simulink library "Enrg_conv_El_to_Mec_Bosch"  (R2016a)
settings: Solver=ode1  StartTime=0.0  StopTime=Inf  FixedStep=0.001  RelTol=1e-3
undefined symbols (not defined in the file): drvEmot_RefTqeMOT, FirstDrivenAxle_FirstDrivenAxleNoOfEmot, FMIKit, SecondDrivenAxle_SecondDrivenAxleNoOfEmot
libraries: Enrg_conv_El_to_Mec_Bosch x13, Electrical_converter x8
(part 3 of 5)

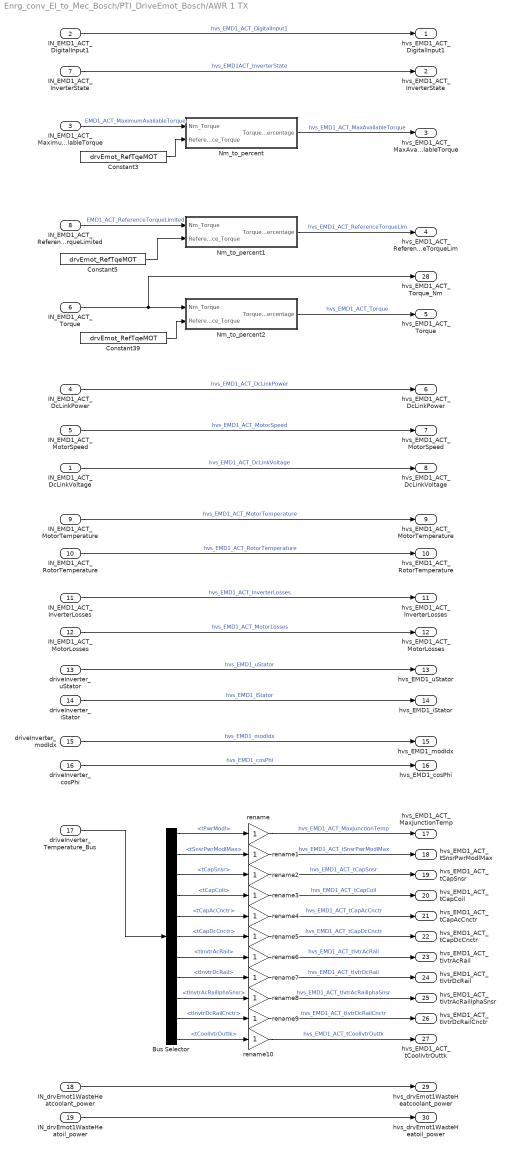
== system Enrg_conv_El_to_Mec_Bosch/PTI_DriveEmot_Bosch/AWR 1 TX ==
  IN_EMD1_ACT_DcLinkVoltage : Inport
  IN_EMD1_ACT_DigitalInput1 : Inport  Port=2
  IN_EMD1_ACT_MaximumAvailableTorque : Inport  Port=3
  IN_EMD1_ACT_DcLinkPower : Inport  Port=4
  IN_EMD1_ACT_MotorSpeed : Inport  Port=5
  IN_EMD1_ACT_Torque : Inport  Port=6
  IN_EMD1_ACT_InverterState : Inport  Port=7
  IN_EMD1_ACT_ReferenceTorqueLimited : Inport  Port=8
  IN_EMD1_ACT_MotorTemperature : Inport  Port=9
  IN_EMD1_ACT_RotorTemperature : Inport  Port=10
  IN_EMD1_ACT_InverterLosses : Inport  Port=11
  IN_EMD1_ACT_MotorLosses : Inport  Port=12
  driveInverter_uStator : Inport  Port=13
  driveInverter_iStator : Inport  Port=14
  driveInverter_modIdx : Inport  Port=15
  driveInverter_cosPhi : Inport  Port=16
  driveInverter_Temperature_Bus : Inport  Port=17
  IN_drvEmot1WasteHeatcoolant_power : Inport  Port=18
  IN_drvEmot1WasteHeatoil_power : Inport  Port=19
  Bus Selector : BusSelector  OutputSignals=tPwrModl,tSnsrPwrModlMax,tCapSnsr,tCapCoil,tCapAcCnctr,tCapDcCnctr,tInvtrAcRail,tInvtrDcRail,tInvtrAcRailIphaSnsr,tInvtrDcRailCnctr,tCoolIvtrOuttk
  Constant3 : Constant  Value=drvEmot_RefTqeMOT
  Constant39 : Constant  Value=drvEmot_RefTqeMOT
  Constant5 : Constant  Value=drvEmot_RefTqeMOT
  Nm_to_percent : Subsystem
  Nm_to_percent1 : Subsystem
  Nm_to_percent2 : Subsystem
  rename{,1..10} (11 alike) : Gain
  hvs_EMD1_ACT_DigitalInput1 : Outport
  hvs_EMD1_ACT_InverterState : Outport  Port=2
  hvs_EMD1_ACT_MaxAvailableTorque : Outport  Port=3
  hvs_EMD1_ACT_ReferenceTorqueLim : Outport  Port=4
  hvs_EMD1_ACT_Torque : Outport  Port=5
  hvs_EMD1_ACT_DcLinkPower : Outport  Port=6
  hvs_EMD1_ACT_MotorSpeed : Outport  Port=7
  hvs_EMD1_ACT_DcLinkVoltage : Outport  Port=8
  hvs_EMD1_ACT_MotorTemperature : Outport  Port=9
  hvs_EMD1_ACT_RotorTemperature : Outport  Port=10
  hvs_EMD1_ACT_InverterLosses : Outport  Port=11
  hvs_EMD1_ACT_MotorLosses : Outport  Port=12
  hvs_EMD1_uStator : Outport  Port=13
  hvs_EMD1_iStator : Outport  Port=14
  hvs_EMD1_modIdx : Outport  Port=15
  hvs_EMD1_cosPhi : Outport  Port=16
  hvs_EMD1_ACT_MaxJunctionTemp : Outport  Port=17
  hvs_EMD1_ACT_tSnsrPwrModlMax : Outport  Port=18
  hvs_EMD1_ACT_tCapSnsr : Outport  Port=19
  hvs_EMD1_ACT_tCapCoil : Outport  Port=20
  hvs_EMD1_ACT_tCapAcCnctr : Outport  Port=21
  hvs_EMD1_ACT_tCapDcCnctr : Outport  Port=22
  hvs_EMD1_ACT_tIvtrAcRail : Outport  Port=23
  hvs_EMD1_ACT_tIvtrDcRail : Outport  Port=24
  hvs_EMD1_ACT_tIvtrAcRailIphaSnsr : Outport  Port=25
  hvs_EMD1_ACT_tIvtrDcRailCnctr : Outport  Port=26
  hvs_EMD1_ACT_tCoolIvtrOuttk : Outport  Port=27
  hvs_EMD1_ACT_Torque_Nm : Outport  Port=28
  hvs_drvEmot1WasteHeatcoolant_power : Outport  Port=29
  hvs_drvEmot1WasteHeatoil_power : Outport  Port=30
  wires:
  Constant5/1 -> Nm_to_percent1/2(Reference_Torque)
  IN_EMD1_ACT_ReferenceTorqueLimited/1 -> Nm_to_percent1/1(Nm_Torque)  "EMD1_ACT_ReferenceTorqueLimited"
  IN_EMD1_ACT_InverterState/1 -> hvs_EMD1_ACT_InverterState/1  "hvs_EMD1ACT_InverterState"
  IN_EMD1_ACT_DcLinkPower/1 -> hvs_EMD1_ACT_DcLinkPower/1  "hvs_EMD1_ACT_DcLinkPower"
  IN_EMD1_ACT_DcLinkVoltage/1 -> hvs_EMD1_ACT_DcLinkVoltage/1  "hvs_EMD1_ACT_DcLinkVoltage"
  Nm_to_percent/1(Torque_Percentage) -> hvs_EMD1_ACT_MaxAvailableTorque/1  "hvs_EMD1_ACT_MaxAvailableTorque"
  Nm_to_percent1/1(Torque_Percentage) -> hvs_EMD1_ACT_ReferenceTorqueLim/1  "hvs_EMD1_ACT_ReferenceTorqueLim"
  IN_EMD1_ACT_MotorSpeed/1 -> hvs_EMD1_ACT_MotorSpeed/1  "hvs_EMD1_ACT_MotorSpeed"
  IN_EMD1_ACT_Torque/1 -> hvs_EMD1_ACT_Torque_Nm/1, Nm_to_percent2/1(Nm_Torque)
  IN_EMD1_ACT_MotorTemperature/1 -> hvs_EMD1_ACT_MotorTemperature/1  "hvs_EMD1_ACT_MotorTemperature"
  IN_EMD1_ACT_DigitalInput1/1 -> hvs_EMD1_ACT_DigitalInput1/1  "hvs_EMD1_ACT_DigitalInput1"
  IN_EMD1_ACT_MaximumAvailableTorque/1 -> Nm_to_percent/1(Nm_Torque)  "EMD1_ACT_MaximumAvailableTorque"
  Constant3/1 -> Nm_to_percent/2(Reference_Torque)
  Nm_to_percent2/1(Torque_Percentage) -> hvs_EMD1_ACT_Torque/1  "hvs_EMD1_ACT_Torque"
  Constant39/1 -> Nm_to_percent2/2(Reference_Torque)
  IN_EMD1_ACT_InverterLosses/1 -> hvs_EMD1_ACT_InverterLosses/1  "hvs_EMD1_ACT_InverterLosses"
  IN_EMD1_ACT_MotorLosses/1 -> hvs_EMD1_ACT_MotorLosses/1  "hvs_EMD1_ACT_MotorLosses"
  IN_EMD1_ACT_RotorTemperature/1 -> hvs_EMD1_ACT_RotorTemperature/1  "hvs_EMD1_ACT_RotorTemperature"
  driveInverter_uStator/1 -> hvs_EMD1_uStator/1  "hvs_EMD1_uStator"
  driveInverter_iStator/1 -> hvs_EMD1_iStator/1  "hvs_EMD1_iStator"
  driveInverter_Temperature_Bus/1 -> Bus Selector/1
  Bus Selector/1 -> rename/1  "<tPwrModl>"
  Bus Selector/2 -> rename1/1  "<tSnsrPwrModlMax>"
  Bus Selector/3 -> rename2/1  "<tCapSnsr>"
  Bus Selector/4 -> rename3/1  "<tCapCoil>"
  Bus Selector/5 -> rename4/1  "<tCapAcCnctr>"
  Bus Selector/6 -> rename5/1  "<tCapDcCnctr>"
  Bus Selector/7 -> rename6/1  "<tInvtrAcRail>"
  Bus Selector/8 -> rename7/1  "<tInvtrDcRail>"
  Bus Selector/9 -> rename8/1  "<tInvtrAcRailIphaSnsr>"
  Bus Selector/10 -> rename9/1  "<tInvtrDcRailCnctr>"
  Bus Selector/11 -> rename10/1  "<tCoolIvtrOuttk>"
  rename/1 -> hvs_EMD1_ACT_MaxJunctionTemp/1  "hvs_EMD1_ACT_MaxJunctionTemp"
  rename1/1 -> hvs_EMD1_ACT_tSnsrPwrModlMax/1  "hvs_EMD1_ACT_tSnsrPwrModlMax"
  rename2/1 -> hvs_EMD1_ACT_tCapSnsr/1  "hvs_EMD1_ACT_tCapSnsr"
  rename3/1 -> hvs_EMD1_ACT_tCapCoil/1  "hvs_EMD1_ACT_tCapCoil"
  rename4/1 -> hvs_EMD1_ACT_tCapAcCnctr/1  "hvs_EMD1_ACT_tCapAcCnctr"
  rename5/1 -> hvs_EMD1_ACT_tCapDcCnctr/1  "hvs_EMD1_ACT_tCapDcCnctr"
  rename6/1 -> hvs_EMD1_ACT_tIvtrAcRail/1  "hvs_EMD1_ACT_tIvtrAcRail"
  rename7/1 -> hvs_EMD1_ACT_tIvtrDcRail/1  "hvs_EMD1_ACT_tIvtrDcRail"
  rename8/1 -> hvs_EMD1_ACT_tIvtrAcRailIphaSnsr/1  "hvs_EMD1_ACT_tIvtrAcRailIphaSnsr"
  rename9/1 -> hvs_EMD1_ACT_tIvtrDcRailCnctr/1  "hvs_EMD1_ACT_tIvtrDcRailCnctr"
  rename10/1 -> hvs_EMD1_ACT_tCoolIvtrOuttk/1  "hvs_EMD1_ACT_tCoolIvtrOuttk"
  driveInverter_modIdx/1 -> hvs_EMD1_modIdx/1  "hvs_EMD1_modIdx"
  driveInverter_cosPhi/1 -> hvs_EMD1_cosPhi/1  "hvs_EMD1_cosPhi"
  IN_drvEmot1WasteHeatcoolant_power/1 -> hvs_drvEmot1WasteHeatcoolant_power/1
  IN_drvEmot1WasteHeatoil_power/1 -> hvs_drvEmot1WasteHeatoil_power/1

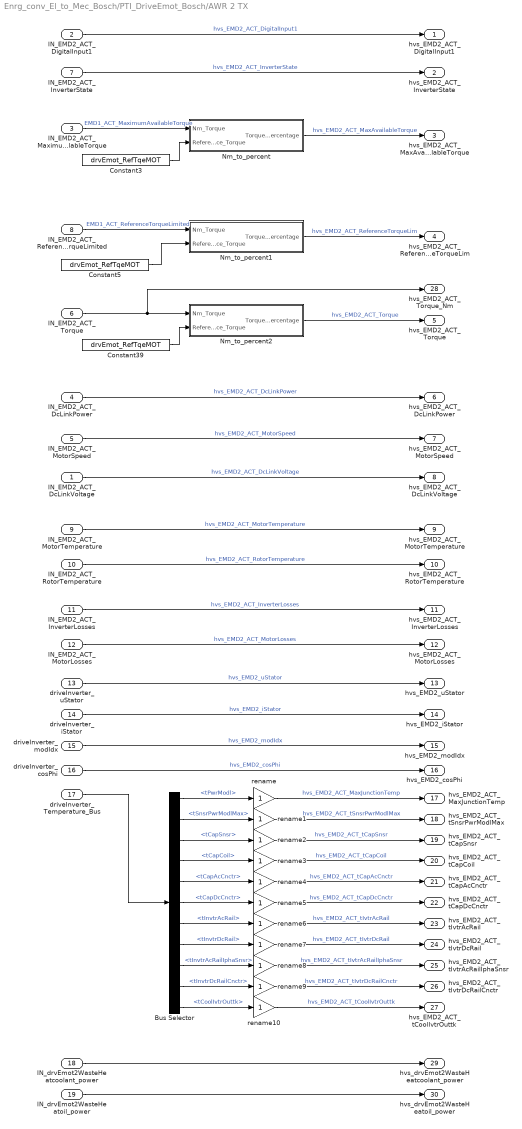
== system Enrg_conv_El_to_Mec_Bosch/PTI_DriveEmot_Bosch/AWR 2 TX ==
  IN_EMD2_ACT_DcLinkVoltage : Inport
  IN_EMD2_ACT_DigitalInput1 : Inport  Port=2
  IN_EMD2_ACT_MaximumAvailableTorque : Inport  Port=3
  IN_EMD2_ACT_DcLinkPower : Inport  Port=4
  IN_EMD2_ACT_MotorSpeed : Inport  Port=5
  IN_EMD2_ACT_Torque : Inport  Port=6
  IN_EMD2_ACT_InverterState : Inport  Port=7
  IN_EMD2_ACT_ReferenceTorqueLimited : Inport  Port=8
  IN_EMD2_ACT_MotorTemperature : Inport  Port=9
  IN_EMD2_ACT_RotorTemperature : Inport  Port=10
  IN_EMD2_ACT_InverterLosses : Inport  Port=11
  IN_EMD2_ACT_MotorLosses : Inport  Port=12
  driveInverter_uStator : Inport  Port=13
  driveInverter_iStator : Inport  Port=14
  driveInverter_modIdx : Inport  Port=15
  driveInverter_cosPhi : Inport  Port=16
  driveInverter_Temperature_Bus : Inport  Port=17
  IN_drvEmot2WasteHeatcoolant_power : Inport  Port=18
  IN_drvEmot2WasteHeatoil_power : Inport  Port=19
  Bus Selector : BusSelector  OutputSignals=tPwrModl,tSnsrPwrModlMax,tCapSnsr,tCapCoil,tCapAcCnctr,tCapDcCnctr,tInvtrAcRail,tInvtrDcRail,tInvtrAcRailIphaSnsr,tInvtrDcRailCnctr,tCoolIvtrOuttk
  Constant3 : Constant  Value=drvEmot_RefTqeMOT
  Constant39 : Constant  Value=drvEmot_RefTqeMOT
  Constant5 : Constant  Value=drvEmot_RefTqeMOT
  Nm_to_percent : Subsystem
  Nm_to_percent1 : Subsystem
  Nm_to_percent2 : Subsystem
  rename{,1..10} (11 alike) : Gain
  hvs_EMD2_ACT_DigitalInput1 : Outport
  hvs_EMD2_ACT_InverterState : Outport  Port=2
  hvs_EMD2_ACT_MaxAvailableTorque : Outport  Port=3
  hvs_EMD2_ACT_ReferenceTorqueLim : Outport  Port=4
  hvs_EMD2_ACT_Torque : Outport  Port=5
  hvs_EMD2_ACT_DcLinkPower : Outport  Port=6
  hvs_EMD2_ACT_MotorSpeed : Outport  Port=7
  hvs_EMD2_ACT_DcLinkVoltage : Outport  Port=8
  hvs_EMD2_ACT_MotorTemperature : Outport  Port=9
  hvs_EMD2_ACT_RotorTemperature : Outport  Port=10
  hvs_EMD2_ACT_InverterLosses : Outport  Port=11
  hvs_EMD2_ACT_MotorLosses : Outport  Port=12
  hvs_EMD2_uStator : Outport  Port=13
  hvs_EMD2_iStator : Outport  Port=14
  hvs_EMD2_modIdx : Outport  Port=15
  hvs_EMD2_cosPhi : Outport  Port=16
  hvs_EMD2_ACT_MaxJunctionTemp : Outport  Port=17
  hvs_EMD2_ACT_tSnsrPwrModlMax : Outport  Port=18
  hvs_EMD2_ACT_tCapSnsr : Outport  Port=19
  hvs_EMD2_ACT_tCapCoil : Outport  Port=20
  hvs_EMD2_ACT_tCapAcCnctr : Outport  Port=21
  hvs_EMD2_ACT_tCapDcCnctr : Outport  Port=22
  hvs_EMD2_ACT_tIvtrAcRail : Outport  Port=23
  hvs_EMD2_ACT_tIvtrDcRail : Outport  Port=24
  hvs_EMD2_ACT_tIvtrAcRailIphaSnsr : Outport  Port=25
  hvs_EMD2_ACT_tIvtrDcRailCnctr : Outport  Port=26
  hvs_EMD2_ACT_tCoolIvtrOuttk : Outport  Port=27
  hvs_EMD2_ACT_Torque_Nm : Outport  Port=28
  hvs_drvEmot2WasteHeatcoolant_power : Outport  Port=29
  hvs_drvEmot2WasteHeatoil_power : Outport  Port=30
  wires:
  Constant5/1 -> Nm_to_percent1/2(Reference_Torque)
  IN_EMD2_ACT_ReferenceTorqueLimited/1 -> Nm_to_percent1/1(Nm_Torque)  "EMD1_ACT_ReferenceTorqueLimited"
  IN_EMD2_ACT_InverterState/1 -> hvs_EMD2_ACT_InverterState/1  "hvs_EMD2_ACT_InverterState"
  IN_EMD2_ACT_DcLinkPower/1 -> hvs_EMD2_ACT_DcLinkPower/1  "hvs_EMD2_ACT_DcLinkPower"
  IN_EMD2_ACT_DcLinkVoltage/1 -> hvs_EMD2_ACT_DcLinkVoltage/1  "hvs_EMD2_ACT_DcLinkVoltage"
  Nm_to_percent/1(Torque_Percentage) -> hvs_EMD2_ACT_MaxAvailableTorque/1  "hvs_EMD2_ACT_MaxAvailableTorque"
  Nm_to_percent1/1(Torque_Percentage) -> hvs_EMD2_ACT_ReferenceTorqueLim/1  "hvs_EMD2_ACT_ReferenceTorqueLim"
  IN_EMD2_ACT_MotorSpeed/1 -> hvs_EMD2_ACT_MotorSpeed/1  "hvs_EMD2_ACT_MotorSpeed"
  IN_EMD2_ACT_Torque/1 -> hvs_EMD2_ACT_Torque_Nm/1, Nm_to_percent2/1(Nm_Torque)
  IN_EMD2_ACT_MotorTemperature/1 -> hvs_EMD2_ACT_MotorTemperature/1  "hvs_EMD2_ACT_MotorTemperature"
  IN_EMD2_ACT_DigitalInput1/1 -> hvs_EMD2_ACT_DigitalInput1/1  "hvs_EMD2_ACT_DigitalInput1"
  IN_EMD2_ACT_MaximumAvailableTorque/1 -> Nm_to_percent/1(Nm_Torque)  "EMD1_ACT_MaximumAvailableTorque"
  Constant3/1 -> Nm_to_percent/2(Reference_Torque)
  Nm_to_percent2/1(Torque_Percentage) -> hvs_EMD2_ACT_Torque/1  "hvs_EMD2_ACT_Torque"
  Constant39/1 -> Nm_to_percent2/2(Reference_Torque)
  IN_EMD2_ACT_InverterLosses/1 -> hvs_EMD2_ACT_InverterLosses/1  "hvs_EMD2_ACT_InverterLosses"
  IN_EMD2_ACT_MotorLosses/1 -> hvs_EMD2_ACT_MotorLosses/1  "hvs_EMD2_ACT_MotorLosses"
  IN_EMD2_ACT_RotorTemperature/1 -> hvs_EMD2_ACT_RotorTemperature/1  "hvs_EMD2_ACT_RotorTemperature"
  driveInverter_uStator/1 -> hvs_EMD2_uStator/1  "hvs_EMD2_uStator"
  driveInverter_iStator/1 -> hvs_EMD2_iStator/1  "hvs_EMD2_iStator"
  driveInverter_Temperature_Bus/1 -> Bus Selector/1
  Bus Selector/1 -> rename/1  "<tPwrModl>"
  Bus Selector/2 -> rename1/1  "<tSnsrPwrModlMax>"
  Bus Selector/3 -> rename2/1  "<tCapSnsr>"
  Bus Selector/4 -> rename3/1  "<tCapCoil>"
  Bus Selector/5 -> rename4/1  "<tCapAcCnctr>"
  Bus Selector/6 -> rename5/1  "<tCapDcCnctr>"
  Bus Selector/7 -> rename6/1  "<tInvtrAcRail>"
  Bus Selector/8 -> rename7/1  "<tInvtrDcRail>"
  Bus Selector/9 -> rename8/1  "<tInvtrAcRailIphaSnsr>"
  Bus Selector/10 -> rename9/1  "<tInvtrDcRailCnctr>"
  Bus Selector/11 -> rename10/1  "<tCoolIvtrOuttk>"
  rename/1 -> hvs_EMD2_ACT_MaxJunctionTemp/1  "hvs_EMD2_ACT_MaxJunctionTemp"
  rename1/1 -> hvs_EMD2_ACT_tSnsrPwrModlMax/1  "hvs_EMD2_ACT_tSnsrPwrModlMax"
  rename2/1 -> hvs_EMD2_ACT_tCapSnsr/1  "hvs_EMD2_ACT_tCapSnsr"
  rename3/1 -> hvs_EMD2_ACT_tCapCoil/1  "hvs_EMD2_ACT_tCapCoil"
  rename4/1 -> hvs_EMD2_ACT_tCapAcCnctr/1  "hvs_EMD2_ACT_tCapAcCnctr"
  rename5/1 -> hvs_EMD2_ACT_tCapDcCnctr/1  "hvs_EMD2_ACT_tCapDcCnctr"
  rename6/1 -> hvs_EMD2_ACT_tIvtrAcRail/1  "hvs_EMD2_ACT_tIvtrAcRail"
  rename7/1 -> hvs_EMD2_ACT_tIvtrDcRail/1  "hvs_EMD2_ACT_tIvtrDcRail"
  rename8/1 -> hvs_EMD2_ACT_tIvtrAcRailIphaSnsr/1  "hvs_EMD2_ACT_tIvtrAcRailIphaSnsr"
  rename9/1 -> hvs_EMD2_ACT_tIvtrDcRailCnctr/1  "hvs_EMD2_ACT_tIvtrDcRailCnctr"
  rename10/1 -> hvs_EMD2_ACT_tCoolIvtrOuttk/1  "hvs_EMD2_ACT_tCoolIvtrOuttk"
  driveInverter_modIdx/1 -> hvs_EMD2_modIdx/1  "hvs_EMD2_modIdx"
  driveInverter_cosPhi/1 -> hvs_EMD2_cosPhi/1  "hvs_EMD2_cosPhi"
  IN_drvEmot2WasteHeatcoolant_power/1 -> hvs_drvEmot2WasteHeatcoolant_power/1
  IN_drvEmot2WasteHeatoil_power/1 -> hvs_drvEmot2WasteHeatoil_power/1

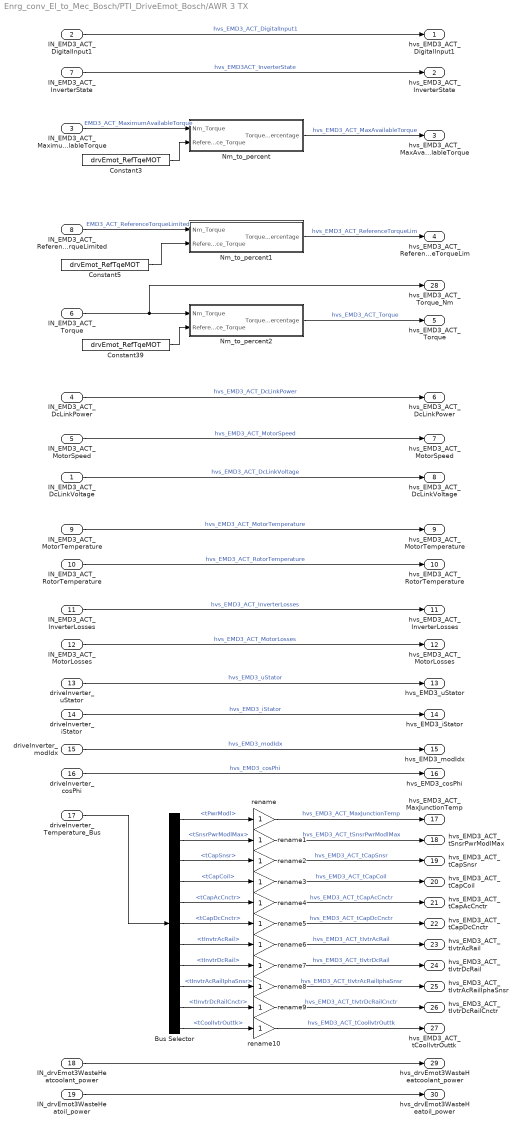
== system Enrg_conv_El_to_Mec_Bosch/PTI_DriveEmot_Bosch/AWR 3 TX ==
  IN_EMD3_ACT_DcLinkVoltage : Inport
  IN_EMD3_ACT_DigitalInput1 : Inport  Port=2
  IN_EMD3_ACT_MaximumAvailableTorque : Inport  Port=3
  IN_EMD3_ACT_DcLinkPower : Inport  Port=4
  IN_EMD3_ACT_MotorSpeed : Inport  Port=5
  IN_EMD3_ACT_Torque : Inport  Port=6
  IN_EMD3_ACT_InverterState : Inport  Port=7
  IN_EMD3_ACT_ReferenceTorqueLimited : Inport  Port=8
  IN_EMD3_ACT_MotorTemperature : Inport  Port=9
  IN_EMD3_ACT_RotorTemperature : Inport  Port=10
  IN_EMD3_ACT_InverterLosses : Inport  Port=11
  IN_EMD3_ACT_MotorLosses : Inport  Port=12
  driveInverter_uStator : Inport  Port=13
  driveInverter_iStator : Inport  Port=14
  driveInverter_modIdx : Inport  Port=15
  driveInverter_cosPhi : Inport  Port=16
  driveInverter_Temperature_Bus : Inport  Port=17
  IN_drvEmot3WasteHeatcoolant_power : Inport  Port=18
  IN_drvEmot3WasteHeatoil_power : Inport  Port=19
  Bus Selector : BusSelector  OutputSignals=tPwrModl,tSnsrPwrModlMax,tCapSnsr,tCapCoil,tCapAcCnctr,tCapDcCnctr,tInvtrAcRail,tInvtrDcRail,tInvtrAcRailIphaSnsr,tInvtrDcRailCnctr,tCoolIvtrOuttk
  Constant3 : Constant  Value=drvEmot_RefTqeMOT
  Constant39 : Constant  Value=drvEmot_RefTqeMOT
  Constant5 : Constant  Value=drvEmot_RefTqeMOT
  Nm_to_percent : Subsystem
  Nm_to_percent1 : Subsystem
  Nm_to_percent2 : Subsystem
  rename{,1..10} (11 alike) : Gain
  hvs_EMD3_ACT_DigitalInput1 : Outport
  hvs_EMD3_ACT_InverterState : Outport  Port=2
  hvs_EMD3_ACT_MaxAvailableTorque : Outport  Port=3
  hvs_EMD3_ACT_ReferenceTorqueLim : Outport  Port=4
  hvs_EMD3_ACT_Torque : Outport  Port=5
  hvs_EMD3_ACT_DcLinkPower : Outport  Port=6
  hvs_EMD3_ACT_MotorSpeed : Outport  Port=7
  hvs_EMD3_ACT_DcLinkVoltage : Outport  Port=8
  hvs_EMD3_ACT_MotorTemperature : Outport  Port=9
  hvs_EMD3_ACT_RotorTemperature : Outport  Port=10
  hvs_EMD3_ACT_InverterLosses : Outport  Port=11
  hvs_EMD3_ACT_MotorLosses : Outport  Port=12
  hvs_EMD3_uStator : Outport  Port=13
  hvs_EMD3_iStator : Outport  Port=14
  hvs_EMD3_modIdx : Outport  Port=15
  hvs_EMD3_cosPhi : Outport  Port=16
  hvs_EMD3_ACT_MaxJunctionTemp : Outport  Port=17
  hvs_EMD3_ACT_tSnsrPwrModlMax : Outport  Port=18
  hvs_EMD3_ACT_tCapSnsr : Outport  Port=19
  hvs_EMD3_ACT_tCapCoil : Outport  Port=20
  hvs_EMD3_ACT_tCapAcCnctr : Outport  Port=21
  hvs_EMD3_ACT_tCapDcCnctr : Outport  Port=22
  hvs_EMD3_ACT_tIvtrAcRail : Outport  Port=23
  hvs_EMD3_ACT_tIvtrDcRail : Outport  Port=24
  hvs_EMD3_ACT_tIvtrAcRailIphaSnsr : Outport  Port=25
  hvs_EMD3_ACT_tIvtrDcRailCnctr : Outport  Port=26
  hvs_EMD3_ACT_tCoolIvtrOuttk : Outport  Port=27
  hvs_EMD3_ACT_Torque_Nm : Outport  Port=28
  hvs_drvEmot3WasteHeatcoolant_power : Outport  Port=29
  hvs_drvEmot3WasteHeatoil_power : Outport  Port=30
  wires:
  rename10/1 -> hvs_EMD3_ACT_tCoolIvtrOuttk/1  "hvs_EMD3_ACT_tCoolIvtrOuttk"
  rename9/1 -> hvs_EMD3_ACT_tIvtrDcRailCnctr/1  "hvs_EMD3_ACT_tIvtrDcRailCnctr"
  rename8/1 -> hvs_EMD3_ACT_tIvtrAcRailIphaSnsr/1  "hvs_EMD3_ACT_tIvtrAcRailIphaSnsr"
  rename7/1 -> hvs_EMD3_ACT_tIvtrDcRail/1  "hvs_EMD3_ACT_tIvtrDcRail"
  rename6/1 -> hvs_EMD3_ACT_tIvtrAcRail/1  "hvs_EMD3_ACT_tIvtrAcRail"
  rename5/1 -> hvs_EMD3_ACT_tCapDcCnctr/1  "hvs_EMD3_ACT_tCapDcCnctr"
  rename4/1 -> hvs_EMD3_ACT_tCapAcCnctr/1  "hvs_EMD3_ACT_tCapAcCnctr"
  rename3/1 -> hvs_EMD3_ACT_tCapCoil/1  "hvs_EMD3_ACT_tCapCoil"
  rename2/1 -> hvs_EMD3_ACT_tCapSnsr/1  "hvs_EMD3_ACT_tCapSnsr"
  rename1/1 -> hvs_EMD3_ACT_tSnsrPwrModlMax/1  "hvs_EMD3_ACT_tSnsrPwrModlMax"
  rename/1 -> hvs_EMD3_ACT_MaxJunctionTemp/1  "hvs_EMD3_ACT_MaxJunctionTemp"
  Bus Selector/11 -> rename10/1  "<tCoolIvtrOuttk>"
  Bus Selector/10 -> rename9/1  "<tInvtrDcRailCnctr>"
  Bus Selector/9 -> rename8/1  "<tInvtrAcRailIphaSnsr>"
  Bus Selector/8 -> rename7/1  "<tInvtrDcRail>"
  Bus Selector/7 -> rename6/1  "<tInvtrAcRail>"
  Bus Selector/6 -> rename5/1  "<tCapDcCnctr>"
  Bus Selector/5 -> rename4/1  "<tCapAcCnctr>"
  Bus Selector/4 -> rename3/1  "<tCapCoil>"
  Bus Selector/3 -> rename2/1  "<tCapSnsr>"
  Bus Selector/2 -> rename1/1  "<tSnsrPwrModlMax>"
  Bus Selector/1 -> rename/1  "<tPwrModl>"
  driveInverter_Temperature_Bus/1 -> Bus Selector/1
  driveInverter_iStator/1 -> hvs_EMD3_iStator/1  "hvs_EMD3_iStator"
  driveInverter_uStator/1 -> hvs_EMD3_uStator/1  "hvs_EMD3_uStator"
  IN_EMD3_ACT_RotorTemperature/1 -> hvs_EMD3_ACT_RotorTemperature/1  "hvs_EMD3_ACT_RotorTemperature"
  IN_EMD3_ACT_MotorLosses/1 -> hvs_EMD3_ACT_MotorLosses/1  "hvs_EMD3_ACT_MotorLosses"
  IN_EMD3_ACT_InverterLosses/1 -> hvs_EMD3_ACT_InverterLosses/1  "hvs_EMD3_ACT_InverterLosses"
  Constant39/1 -> Nm_to_percent2/2(Reference_Torque)
  Nm_to_percent2/1(Torque_Percentage) -> hvs_EMD3_ACT_Torque/1  "hvs_EMD3_ACT_Torque"
  Constant3/1 -> Nm_to_percent/2(Reference_Torque)
  IN_EMD3_ACT_MaximumAvailableTorque/1 -> Nm_to_percent/1(Nm_Torque)  "EMD3_ACT_MaximumAvailableTorque"
  IN_EMD3_ACT_DigitalInput1/1 -> hvs_EMD3_ACT_DigitalInput1/1  "hvs_EMD3_ACT_DigitalInput1"
  IN_EMD3_ACT_MotorTemperature/1 -> hvs_EMD3_ACT_MotorTemperature/1  "hvs_EMD3_ACT_MotorTemperature"
  IN_EMD3_ACT_Torque/1 -> hvs_EMD3_ACT_Torque_Nm/1, Nm_to_percent2/1(Nm_Torque)
  IN_EMD3_ACT_MotorSpeed/1 -> hvs_EMD3_ACT_MotorSpeed/1  "hvs_EMD3_ACT_MotorSpeed"
  Nm_to_percent1/1(Torque_Percentage) -> hvs_EMD3_ACT_ReferenceTorqueLim/1  "hvs_EMD3_ACT_ReferenceTorqueLim"
  Nm_to_percent/1(Torque_Percentage) -> hvs_EMD3_ACT_MaxAvailableTorque/1  "hvs_EMD3_ACT_MaxAvailableTorque"
  IN_EMD3_ACT_DcLinkVoltage/1 -> hvs_EMD3_ACT_DcLinkVoltage/1  "hvs_EMD3_ACT_DcLinkVoltage"
  IN_EMD3_ACT_DcLinkPower/1 -> hvs_EMD3_ACT_DcLinkPower/1  "hvs_EMD3_ACT_DcLinkPower"
  IN_EMD3_ACT_InverterState/1 -> hvs_EMD3_ACT_InverterState/1  "hvs_EMD3ACT_InverterState"
  IN_EMD3_ACT_ReferenceTorqueLimited/1 -> Nm_to_percent1/1(Nm_Torque)  "EMD3_ACT_ReferenceTorqueLimited"
  Constant5/1 -> Nm_to_percent1/2(Reference_Torque)
  driveInverter_modIdx/1 -> hvs_EMD3_modIdx/1  "hvs_EMD3_modIdx"
  driveInverter_cosPhi/1 -> hvs_EMD3_cosPhi/1  "hvs_EMD3_cosPhi"
  IN_drvEmot3WasteHeatcoolant_power/1 -> hvs_drvEmot3WasteHeatcoolant_power/1
  IN_drvEmot3WasteHeatoil_power/1 -> hvs_drvEmot3WasteHeatoil_power/1

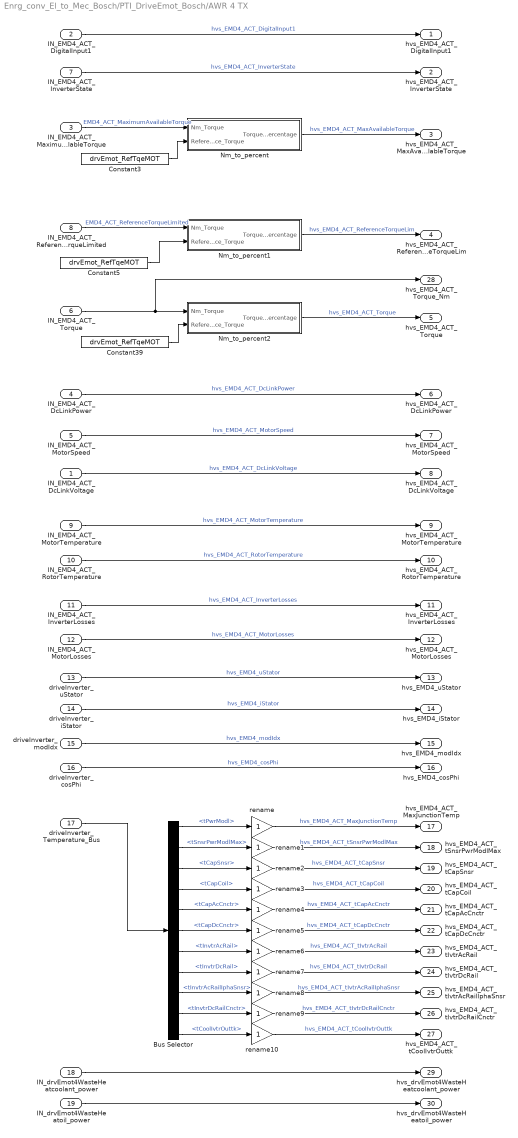
== system Enrg_conv_El_to_Mec_Bosch/PTI_DriveEmot_Bosch/AWR 4 TX ==
  IN_EMD4_ACT_DcLinkVoltage : Inport
  IN_EMD4_ACT_DigitalInput1 : Inport  Port=2
  IN_EMD4_ACT_MaximumAvailableTorque : Inport  Port=3
  IN_EMD4_ACT_DcLinkPower : Inport  Port=4
  IN_EMD4_ACT_MotorSpeed : Inport  Port=5
  IN_EMD4_ACT_Torque : Inport  Port=6
  IN_EMD4_ACT_InverterState : Inport  Port=7
  IN_EMD4_ACT_ReferenceTorqueLimited : Inport  Port=8
  IN_EMD4_ACT_MotorTemperature : Inport  Port=9
  IN_EMD4_ACT_RotorTemperature : Inport  Port=10
  IN_EMD4_ACT_InverterLosses : Inport  Port=11
  IN_EMD4_ACT_MotorLosses : Inport  Port=12
  driveInverter_uStator : Inport  Port=13
  driveInverter_iStator : Inport  Port=14
  driveInverter_modIdx : Inport  Port=15
  driveInverter_cosPhi : Inport  Port=16
  driveInverter_Temperature_Bus : Inport  Port=17
  IN_drvEmot4WasteHeatcoolant_power : Inport  Port=18
  IN_drvEmot4WasteHeatoil_power : Inport  Port=19
  Bus Selector : BusSelector  OutputSignals=tPwrModl,tSnsrPwrModlMax,tCapSnsr,tCapCoil,tCapAcCnctr,tCapDcCnctr,tInvtrAcRail,tInvtrDcRail,tInvtrAcRailIphaSnsr,tInvtrDcRailCnctr,tCoolIvtrOuttk
  Constant3 : Constant  Value=drvEmot_RefTqeMOT
  Constant39 : Constant  Value=drvEmot_RefTqeMOT
  Constant5 : Constant  Value=drvEmot_RefTqeMOT
  Nm_to_percent : Subsystem
  Nm_to_percent1 : Subsystem
  Nm_to_percent2 : Subsystem
  rename{,1..10} (11 alike) : Gain
  hvs_EMD4_ACT_DigitalInput1 : Outport
  hvs_EMD4_ACT_InverterState : Outport  Port=2
  hvs_EMD4_ACT_MaxAvailableTorque : Outport  Port=3
  hvs_EMD4_ACT_ReferenceTorqueLim : Outport  Port=4
  hvs_EMD4_ACT_Torque : Outport  Port=5
  hvs_EMD4_ACT_DcLinkPower : Outport  Port=6
  hvs_EMD4_ACT_MotorSpeed : Outport  Port=7
  hvs_EMD4_ACT_DcLinkVoltage : Outport  Port=8
  hvs_EMD4_ACT_MotorTemperature : Outport  Port=9
  hvs_EMD4_ACT_RotorTemperature : Outport  Port=10
  hvs_EMD4_ACT_InverterLosses : Outport  Port=11
  hvs_EMD4_ACT_MotorLosses : Outport  Port=12
  hvs_EMD4_uStator : Outport  Port=13
  hvs_EMD4_iStator : Outport  Port=14
  hvs_EMD4_modIdx : Outport  Port=15
  hvs_EMD4_cosPhi : Outport  Port=16
  hvs_EMD4_ACT_MaxJunctionTemp : Outport  Port=17
  hvs_EMD4_ACT_tSnsrPwrModlMax : Outport  Port=18
  hvs_EMD4_ACT_tCapSnsr : Outport  Port=19
  hvs_EMD4_ACT_tCapCoil : Outport  Port=20
  hvs_EMD4_ACT_tCapAcCnctr : Outport  Port=21
  hvs_EMD4_ACT_tCapDcCnctr : Outport  Port=22
  hvs_EMD4_ACT_tIvtrAcRail : Outport  Port=23
  hvs_EMD4_ACT_tIvtrDcRail : Outport  Port=24
  hvs_EMD4_ACT_tIvtrAcRailIphaSnsr : Outport  Port=25
  hvs_EMD4_ACT_tIvtrDcRailCnctr : Outport  Port=26
  hvs_EMD4_ACT_tCoolIvtrOuttk : Outport  Port=27
  hvs_EMD4_ACT_Torque_Nm : Outport  Port=28
  hvs_drvEmot4WasteHeatcoolant_power : Outport  Port=29
  hvs_drvEmot4WasteHeatoil_power : Outport  Port=30
  wires:
  rename10/1 -> hvs_EMD4_ACT_tCoolIvtrOuttk/1  "hvs_EMD4_ACT_tCoolIvtrOuttk"
  rename9/1 -> hvs_EMD4_ACT_tIvtrDcRailCnctr/1  "hvs_EMD4_ACT_tIvtrDcRailCnctr"
  rename8/1 -> hvs_EMD4_ACT_tIvtrAcRailIphaSnsr/1  "hvs_EMD4_ACT_tIvtrAcRailIphaSnsr"
  rename7/1 -> hvs_EMD4_ACT_tIvtrDcRail/1  "hvs_EMD4_ACT_tIvtrDcRail"
  rename6/1 -> hvs_EMD4_ACT_tIvtrAcRail/1  "hvs_EMD4_ACT_tIvtrAcRail"
  rename5/1 -> hvs_EMD4_ACT_tCapDcCnctr/1  "hvs_EMD4_ACT_tCapDcCnctr"
  rename4/1 -> hvs_EMD4_ACT_tCapAcCnctr/1  "hvs_EMD4_ACT_tCapAcCnctr"
  rename3/1 -> hvs_EMD4_ACT_tCapCoil/1  "hvs_EMD4_ACT_tCapCoil"
  rename2/1 -> hvs_EMD4_ACT_tCapSnsr/1  "hvs_EMD4_ACT_tCapSnsr"
  rename1/1 -> hvs_EMD4_ACT_tSnsrPwrModlMax/1  "hvs_EMD4_ACT_tSnsrPwrModlMax"
  rename/1 -> hvs_EMD4_ACT_MaxJunctionTemp/1  "hvs_EMD4_ACT_MaxJunctionTemp"
  Bus Selector/11 -> rename10/1  "<tCoolIvtrOuttk>"
  Bus Selector/10 -> rename9/1  "<tInvtrDcRailCnctr>"
  Bus Selector/9 -> rename8/1  "<tInvtrAcRailIphaSnsr>"
  Bus Selector/8 -> rename7/1  "<tInvtrDcRail>"
  Bus Selector/7 -> rename6/1  "<tInvtrAcRail>"
  Bus Selector/6 -> rename5/1  "<tCapDcCnctr>"
  Bus Selector/5 -> rename4/1  "<tCapAcCnctr>"
  Bus Selector/4 -> rename3/1  "<tCapCoil>"
  Bus Selector/3 -> rename2/1  "<tCapSnsr>"
  Bus Selector/2 -> rename1/1  "<tSnsrPwrModlMax>"
  Bus Selector/1 -> rename/1  "<tPwrModl>"
  driveInverter_Temperature_Bus/1 -> Bus Selector/1
  driveInverter_iStator/1 -> hvs_EMD4_iStator/1  "hvs_EMD4_iStator"
  driveInverter_uStator/1 -> hvs_EMD4_uStator/1  "hvs_EMD4_uStator"
  IN_EMD4_ACT_RotorTemperature/1 -> hvs_EMD4_ACT_RotorTemperature/1  "hvs_EMD4_ACT_RotorTemperature"
  IN_EMD4_ACT_MotorLosses/1 -> hvs_EMD4_ACT_MotorLosses/1  "hvs_EMD4_ACT_MotorLosses"
  IN_EMD4_ACT_InverterLosses/1 -> hvs_EMD4_ACT_InverterLosses/1  "hvs_EMD4_ACT_InverterLosses"
  Constant39/1 -> Nm_to_percent2/2(Reference_Torque)
  Nm_to_percent2/1(Torque_Percentage) -> hvs_EMD4_ACT_Torque/1  "hvs_EMD4_ACT_Torque"
  Constant3/1 -> Nm_to_percent/2(Reference_Torque)
  IN_EMD4_ACT_MaximumAvailableTorque/1 -> Nm_to_percent/1(Nm_Torque)  "EMD4_ACT_MaximumAvailableTorque"
  IN_EMD4_ACT_DigitalInput1/1 -> hvs_EMD4_ACT_DigitalInput1/1  "hvs_EMD4_ACT_DigitalInput1"
  IN_EMD4_ACT_MotorTemperature/1 -> hvs_EMD4_ACT_MotorTemperature/1  "hvs_EMD4_ACT_MotorTemperature"
  IN_EMD4_ACT_Torque/1 -> hvs_EMD4_ACT_Torque_Nm/1, Nm_to_percent2/1(Nm_Torque)
  IN_EMD4_ACT_MotorSpeed/1 -> hvs_EMD4_ACT_MotorSpeed/1  "hvs_EMD4_ACT_MotorSpeed"
  Nm_to_percent1/1(Torque_Percentage) -> hvs_EMD4_ACT_ReferenceTorqueLim/1  "hvs_EMD4_ACT_ReferenceTorqueLim"
  Nm_to_percent/1(Torque_Percentage) -> hvs_EMD4_ACT_MaxAvailableTorque/1  "hvs_EMD4_ACT_MaxAvailableTorque"
  IN_EMD4_ACT_DcLinkVoltage/1 -> hvs_EMD4_ACT_DcLinkVoltage/1  "hvs_EMD4_ACT_DcLinkVoltage"
  IN_EMD4_ACT_DcLinkPower/1 -> hvs_EMD4_ACT_DcLinkPower/1  "hvs_EMD4_ACT_DcLinkPower"
  IN_EMD4_ACT_InverterState/1 -> hvs_EMD4_ACT_InverterState/1  "hvs_EMD4_ACT_InverterState"
  IN_EMD4_ACT_ReferenceTorqueLimited/1 -> Nm_to_percent1/1(Nm_Torque)  "EMD4_ACT_ReferenceTorqueLimited"
  Constant5/1 -> Nm_to_percent1/2(Reference_Torque)
  driveInverter_modIdx/1 -> hvs_EMD4_modIdx/1  "hvs_EMD4_modIdx"
  driveInverter_cosPhi/1 -> hvs_EMD4_cosPhi/1  "hvs_EMD4_cosPhi"
  IN_drvEmot4WasteHeatcoolant_power/1 -> hvs_drvEmot4WasteHeatcoolant_power/1
  IN_drvEmot4WasteHeatoil_power/1 -> hvs_drvEmot4WasteHeatoil_power/1

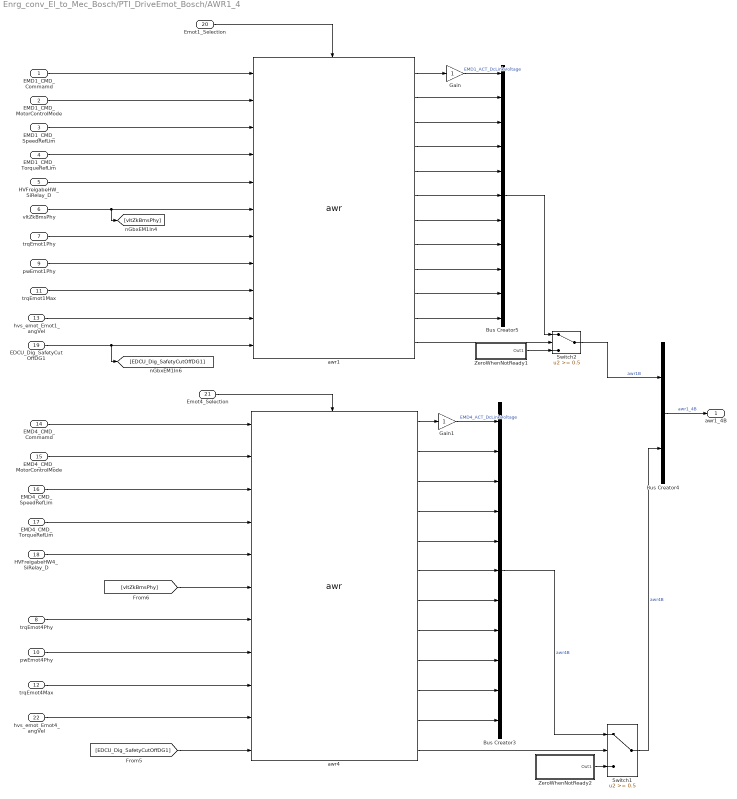
== system Enrg_conv_El_to_Mec_Bosch/PTI_DriveEmot_Bosch/AWR1_4 ==
  EMD1_CMD_Commamd : Inport
  EMD1_CMD_MotorControlMode : Inport  Port=2
  EMD1_CMD_SpeedRefLim : Inport  Port=3
  EMD1_CMD_TorqueRefLim : Inport  Port=4
  HVFreigabeHW_SiRelay_D : Inport  Port=5
  vltZkBmsPhy : Inport  Port=6
  trqEmot1Phy : Inport  Port=7
  trqEmot4Phy : Inport  Port=8
  pwEmot1Phy : Inport  Port=9
  pwEmot4Phy : Inport  Port=10
  trqEmot1Max : Inport  Port=11
  trqEmot4Max : Inport  Port=12
  hvs_emot_Emot1_angVel : Inport  Port=13
  EMD4_CMD_Commamd : Inport  Port=14
  EMD4_CMD_MotorControlMode : Inport  Port=15
  EMD4_CMD_SpeedRefLim : Inport  Port=16
  EMD4_CMD_TorqueRefLim : Inport  Port=17
  HVFreigabeHW4_SiRelay_D : Inport  Port=18
  EDCU_Dig_SafetyCutOffDG1 : Inport  Port=19
  Emot1_Selection : Inport  Port=20
  Emot4_Selection : Inport  Port=21
  hvs_emot_Emot4_angVel : Inport  Port=22
  Bus Creator3 : BusCreator  Inputs=11
  Bus Creator4 : BusCreator  Inputs=2
  Bus Creator5 : BusCreator  Inputs=11
  Gain : Gain
  Gain1 : Gain
  Switch1 : Switch  Threshold=0.5
  Switch2 : Switch  Threshold=0.5
  ZeroWhenNotReady1 : Subsystem  TreatAsAtomicUnit=on
  ZeroWhenNotReady2 : Subsystem  TreatAsAtomicUnit=on
  awr1 : Electrical_converter/awr  SystemSampleTime=-1
  awr4 : Electrical_converter/awr  SystemSampleTime=-1
  awr1_4B : Outport
  wires:
  hvs_emot_Emot1_angVel/1 -> awr1/10
  vltZkBmsPhy/1 -> [vltZkBmsPhy], awr1/6
  EMD1_CMD_MotorControlMode/1 -> awr1/2
  EMD4_CMD_MotorControlMode/1 -> awr4/2
  hvs_emot_Emot4_angVel/1 -> awr4/10
  Gain1/1 -> Bus Creator3/1  "EMD4_ACT_DcLinkVoltage"
  Gain/1 -> Bus Creator5/1  "EMD1_ACT_DcLinkVoltage"
  EMD1_CMD_SpeedRefLim/1 -> awr1/3
  EMD1_CMD_TorqueRefLim/1 -> awr1/4
  HVFreigabeHW_SiRelay_D/1 -> awr1/5
  HVFreigabeHW4_SiRelay_D/1 -> awr4/5
  EMD4_CMD_SpeedRefLim/1 -> awr4/3
  EMD4_CMD_Commamd/1 -> awr4/1
  EMD4_CMD_TorqueRefLim/1 -> awr4/4
  Bus Creator4/1 -> awr1_4B/1  "awr1_4B"
  trqEmot4Phy/1 -> awr4/7
  pwEmot4Phy/1 -> awr4/8
  trqEmot4Max/1 -> awr4/9
  trqEmot1Phy/1 -> awr1/7
  pwEmot1Phy/1 -> awr1/8
  trqEmot1Max/1 -> awr1/9
  Bus Creator3/1 -> Switch1/1  "awr4B"
  ZeroWhenNotReady2/1(Out1) -> Switch1/3
  Switch1/1 -> Bus Creator4/2  "awr4B"
  awr4/2 -> Bus Creator3/2
  awr4/3 -> Bus Creator3/3
  awr4/10 -> Bus Creator3/10
  awr4/11 -> Bus Creator3/11
  awr4/5 -> Bus Creator3/5
  awr4/9 -> Bus Creator3/9
  awr4/8 -> Bus Creator3/8
  awr4/7 -> Bus Creator3/7
  awr4/6 -> Bus Creator3/6
  awr4/1 -> Gain1/1
  awr4/4 -> Bus Creator3/4
  ZeroWhenNotReady1/1(Out1) -> Switch2/3
  Switch2/1 -> Bus Creator4/1  "awr1B"
  awr4/12 -> Switch1/2
  awr1/9 -> Bus Creator5/9
  awr1/7 -> Bus Creator5/7
  awr1/6 -> Bus Creator5/6
  awr1/10 -> Bus Creator5/10
  awr1/11 -> Bus Creator5/11
  awr1/8 -> Bus Creator5/8
  awr1/5 -> Bus Creator5/5
  awr1/4 -> Bus Creator5/4
  awr1/1 -> Gain/1
  awr1/3 -> Bus Creator5/3
  awr1/2 -> Bus Creator5/2
  awr1/12 -> Switch2/2
  Bus Creator5/1 -> Switch2/1
  EMD1_CMD_Commamd/1 -> awr1/1
  [vltZkBmsPhy] -> awr4/6
  EDCU_Dig_SafetyCutOffDG1/1 -> [EDCU_Dig_SafetyCutOffDG1], awr1/11
  [EDCU_Dig_SafetyCutOffDG1] -> awr4/11
  Emot4_Selection/1 -> awr4/Enable
  Emot1_Selection/1 -> awr1/Enable

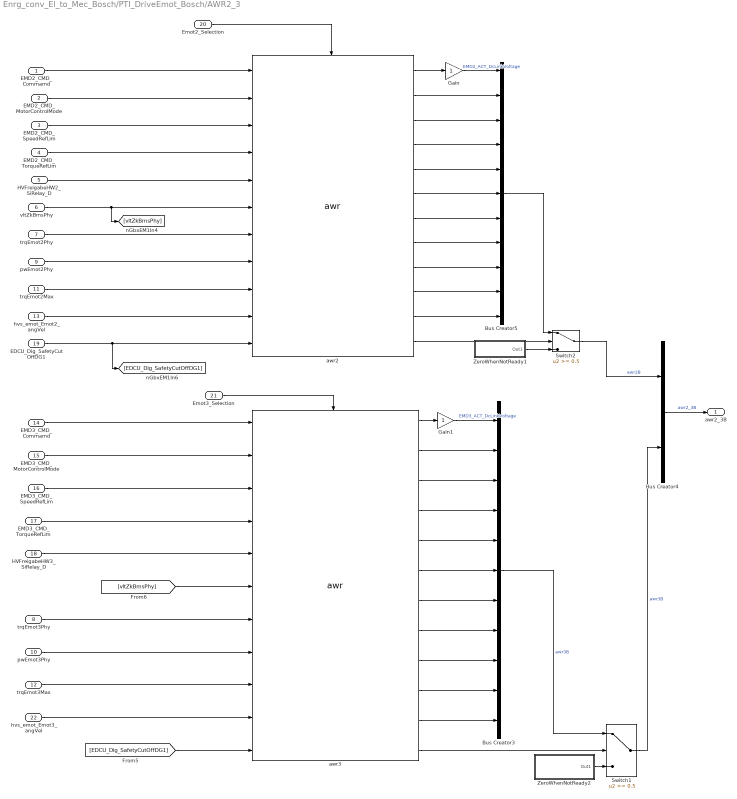
== system Enrg_conv_El_to_Mec_Bosch/PTI_DriveEmot_Bosch/AWR2_3 ==
  EMD2_CMD_Commamd : Inport
  EMD2_CMD_MotorControlMode : Inport  Port=2
  EMD2_CMD_SpeedRefLim : Inport  Port=3
  EMD2_CMD_TorqueRefLim : Inport  Port=4
  HVFreigabeHW2_SiRelay_D : Inport  Port=5
  vltZkBmsPhy : Inport  Port=6
  trqEmot2Phy : Inport  Port=7
  trqEmot3Phy : Inport  Port=8
  pwEmot2Phy : Inport  Port=9
  pwEmot3Phy : Inport  Port=10
  trqEmot2Max : Inport  Port=11
  trqEmot3Max : Inport  Port=12
  hvs_emot_Emot2_angVel : Inport  Port=13
  EMD3_CMD_Commamd : Inport  Port=14
  EMD3_CMD_MotorControlMode : Inport  Port=15
  EMD3_CMD_SpeedRefLim : Inport  Port=16
  EMD3_CMD_TorqueRefLim : Inport  Port=17
  HVFreigabeHW3_SiRelay_D : Inport  Port=18
  EDCU_Dig_SafetyCutOffDG1 : Inport  Port=19
  Emot2_Selection : Inport  Port=20
  Emot3_Selection : Inport  Port=21
  hvs_emot_Emot3_angVel : Inport  Port=22
  Bus Creator3 : BusCreator  Inputs=11
  Bus Creator4 : BusCreator  Inputs=2
  Bus Creator5 : BusCreator  Inputs=11
  Gain : Gain
  Gain1 : Gain
  Switch1 : Switch  Threshold=0.5
  Switch2 : Switch  Threshold=0.5
  ZeroWhenNotReady1 : Subsystem  TreatAsAtomicUnit=on
  ZeroWhenNotReady2 : Subsystem  TreatAsAtomicUnit=on
  awr2 : Electrical_converter/awr  SystemSampleTime=-1
  awr3 : Electrical_converter/awr  SystemSampleTime=-1
  awr2_3B : Outport
  wires:
  [vltZkBmsPhy] -> awr3/6
  EMD2_CMD_Commamd/1 -> awr2/1
  Bus Creator5/1 -> Switch2/1
  awr2/12 -> Switch2/2
  awr2/2 -> Bus Creator5/2
  awr2/3 -> Bus Creator5/3
  awr2/1 -> Gain/1
  awr2/4 -> Bus Creator5/4
  awr2/5 -> Bus Creator5/5
  awr2/8 -> Bus Creator5/8
  awr2/11 -> Bus Creator5/11
  awr2/10 -> Bus Creator5/10
  awr2/6 -> Bus Creator5/6
  awr2/7 -> Bus Creator5/7
  awr2/9 -> Bus Creator5/9
  awr3/12 -> Switch1/2
  Switch2/1 -> Bus Creator4/1  "awr2B"
  ZeroWhenNotReady1/1(Out1) -> Switch2/3
  awr3/4 -> Bus Creator3/4
  awr3/1 -> Gain1/1
  awr3/6 -> Bus Creator3/6
  awr3/7 -> Bus Creator3/7
  awr3/8 -> Bus Creator3/8
  awr3/9 -> Bus Creator3/9
  awr3/5 -> Bus Creator3/5
  awr3/11 -> Bus Creator3/11
  awr3/10 -> Bus Creator3/10
  awr3/3 -> Bus Creator3/3
  awr3/2 -> Bus Creator3/2
  Switch1/1 -> Bus Creator4/2  "awr3B"
  ZeroWhenNotReady2/1(Out1) -> Switch1/3
  Bus Creator3/1 -> Switch1/1  "awr3B"
  trqEmot2Max/1 -> awr2/9
  pwEmot2Phy/1 -> awr2/8
  trqEmot2Phy/1 -> awr2/7
  trqEmot3Max/1 -> awr3/9
  pwEmot3Phy/1 -> awr3/8
  trqEmot3Phy/1 -> awr3/7
  Bus Creator4/1 -> awr2_3B/1  "awr2_3B"
  EMD3_CMD_TorqueRefLim/1 -> awr3/4
  EMD3_CMD_Commamd/1 -> awr3/1
  EMD3_CMD_SpeedRefLim/1 -> awr3/3
  HVFreigabeHW3_SiRelay_D/1 -> awr3/5
  HVFreigabeHW2_SiRelay_D/1 -> awr2/5
  EMD2_CMD_TorqueRefLim/1 -> awr2/4
  EMD2_CMD_SpeedRefLim/1 -> awr2/3
  Gain/1 -> Bus Creator5/1  "EMD2_ACT_DcLinkVoltage"
  Gain1/1 -> Bus Creator3/1  "EMD3_ACT_DcLinkVoltage"
  hvs_emot_Emot3_angVel/1 -> awr3/10
  EMD3_CMD_MotorControlMode/1 -> awr3/2
  EMD2_CMD_MotorControlMode/1 -> awr2/2
  vltZkBmsPhy/1 -> awr2/6, [vltZkBmsPhy]
  hvs_emot_Emot2_angVel/1 -> awr2/10
  EDCU_Dig_SafetyCutOffDG1/1 -> [EDCU_Dig_SafetyCutOffDG1], awr2/11
  [EDCU_Dig_SafetyCutOffDG1] -> awr3/11
  Emot2_Selection/1 -> awr2/Enable
  Emot3_Selection/1 -> awr3/Enable

== system Enrg_conv_El_to_Mec_Bosch/PTI_DriveEmot_Bosch/EMD1_CMD_Command ==
  EMD1_CMD_ClearErrors : Inport
  EMD1_CMD_MotorControlMode : Inport  Port=2
  Compare To Constant : Subsystem  mask(Compare To Constant){relop===, const=1, OutDataTypeStr=boolean, ZeroCross=on}
      mask prompts: relop "Simulink:masks:Operator_MP"; const "Simulink:masks:ConstantValue_MP"; OutDataTypeStr "Simulink:masks:OutputDataType_MP"; ZeroCross "Simulink:masks:EnableZerocrossingDetection_MP"
      mask help: Simulink:masks:CompareToConstant_MD
      mask init:
      | blkName = gcb;
      | 
      | if strcmp(get_param(gcbh,'OutDataTypeStr'),'boolean')
      | 	setValue = 'boolean';
      | else
      | 	setValue = 'fixdt(0, 8)';
      | end
      | 
      | set_param([blkName,'/Compare'],'relop',relop, ...
      | 	'OutDataTypeStr', setValue, 'ZeroCross', ZeroCross);
      | 
      | str = [relop,' C']; %default
      | 
      | const_str = get_param(blkName, 'const');
      | 
      | if isempty(strfind(const_str, ' ')) && isempty(strfind(const_str, ','))
      |     % scalar or single expression
      |     if isempty(str2num(const_str))
      |         %expression
      |         str = [relop, ' ', const_str];
      |     elseif length(const) == 1
      |         str = [relop,' ',num2str(double(const))];
      |     end
      | end
      mask TypeOptions relop: == | ~= | < | <= | >= | >
      mask TypeOptions OutDataTypeStr: Simulink:masks:uint8 | Simulink:masks:boolean
      mask Callback ZeroCross: sl('zeroCrossEnable', gcbh);
      mask Display: disp(str)
  Compare To Constant1 : Subsystem  mask(Compare To Constant){relop===, const=1, OutDataTypeStr=boolean, ZeroCross=on}
      mask prompts: relop "Simulink:masks:Operator_MP"; const "Simulink:masks:ConstantValue_MP"; OutDataTypeStr "Simulink:masks:OutputDataType_MP"; ZeroCross "Simulink:masks:EnableZerocrossingDetection_MP"
      mask help: Simulink:masks:CompareToConstant_MD
      mask init: same as Enrg_conv_El_to_Mec_Bosch/PTI_DriveEmot_Bosch/EMD1_CMD_Command/Compare To Constant
      mask TypeOptions relop: == | ~= | < | <= | >= | >
      mask TypeOptions OutDataTypeStr: Simulink:masks:uint8 | Simulink:masks:boolean
      mask Callback ZeroCross: sl('zeroCrossEnable', gcbh);
      mask Display: disp(str)
  Constant : Constant  Value=4
  Constant3 : Constant
  Constant4 : Constant  Value=0
  Switch : Switch  Threshold=0.5
  Switch1 : Switch  Threshold=0.5
  Out_EMD1_CMD_Command : Outport
  wires:
  Compare To Constant/1(y) -> Switch1/2
  Switch/1 -> Out_EMD1_CMD_Command/1
  Constant4/1 -> Switch1/3
  Constant3/1 -> Switch1/1
  Constant/1 -> Switch/1
  Switch1/1 -> Switch/3
  Compare To Constant1/1(y) -> Switch/2
  EMD1_CMD_ClearErrors/1 -> Compare To Constant1/1(u)
  EMD1_CMD_MotorControlMode/1 -> Compare To Constant/1(u)

== system Enrg_conv_El_to_Mec_Bosch/PTI_DriveEmot_Bosch/EMD1_CMD_Command1 ==
  EMD1_CMD_ClearErrors : Inport
  EMD1_CMD_MotorControlMode : Inport  Port=2
  Compare To Constant : Subsystem  mask(Compare To Constant){relop===, const=1, OutDataTypeStr=boolean, ZeroCross=on}
      mask prompts: relop "Simulink:masks:Operator_MP"; const "Simulink:masks:ConstantValue_MP"; OutDataTypeStr "Simulink:masks:OutputDataType_MP"; ZeroCross "Simulink:masks:EnableZerocrossingDetection_MP"
      mask help: Simulink:masks:CompareToConstant_MD
      mask init: same as Enrg_conv_El_to_Mec_Bosch/PTI_DriveEmot_Bosch/EMD1_CMD_Command/Compare To Constant
      mask TypeOptions relop: == | ~= | < | <= | >= | >
      mask TypeOptions OutDataTypeStr: Simulink:masks:uint8 | Simulink:masks:boolean
      mask Callback ZeroCross: sl('zeroCrossEnable', gcbh);
      mask Display: disp(str)
  Compare To Constant1 : Subsystem  mask(Compare To Constant){relop===, const=1, OutDataTypeStr=boolean, ZeroCross=on}
      mask prompts: relop "Simulink:masks:Operator_MP"; const "Simulink:masks:ConstantValue_MP"; OutDataTypeStr "Simulink:masks:OutputDataType_MP"; ZeroCross "Simulink:masks:EnableZerocrossingDetection_MP"
      mask help: Simulink:masks:CompareToConstant_MD
      mask init: same as Enrg_conv_El_to_Mec_Bosch/PTI_DriveEmot_Bosch/EMD1_CMD_Command/Compare To Constant
      mask TypeOptions relop: == | ~= | < | <= | >= | >
      mask TypeOptions OutDataTypeStr: Simulink:masks:uint8 | Simulink:masks:boolean
      mask Callback ZeroCross: sl('zeroCrossEnable', gcbh);
      mask Display: disp(str)
  Constant : Constant  Value=4
  Constant3 : Constant
  Constant4 : Constant  Value=0
  Switch : Switch  Threshold=0.5
  Switch1 : Switch  Threshold=0.5
  Out_EMD1_CMD_Command : Outport
  wires:
  Compare To Constant/1(y) -> Switch1/2
  Switch/1 -> Out_EMD1_CMD_Command/1
  Constant4/1 -> Switch1/3
  Constant3/1 -> Switch1/1
  Constant/1 -> Switch/1
  Switch1/1 -> Switch/3
  Compare To Constant1/1(y) -> Switch/2
  EMD1_CMD_ClearErrors/1 -> Compare To Constant1/1(u)
  EMD1_CMD_MotorControlMode/1 -> Compare To Constant/1(u)

== system Enrg_conv_El_to_Mec_Bosch/PTI_DriveEmot_Bosch/EMD1_CMD_Command2 ==
  EMD1_CMD_ClearErrors : Inport
  EMD1_CMD_MotorControlMode : Inport  Port=2
  Compare To Constant : Subsystem  mask(Compare To Constant){relop===, const=1, OutDataTypeStr=boolean, ZeroCross=on}
      mask prompts: relop "Simulink:masks:Operator_MP"; const "Simulink:masks:ConstantValue_MP"; OutDataTypeStr "Simulink:masks:OutputDataType_MP"; ZeroCross "Simulink:masks:EnableZerocrossingDetection_MP"
      mask help: Simulink:masks:CompareToConstant_MD
      mask init: same as Enrg_conv_El_to_Mec_Bosch/PTI_DriveEmot_Bosch/EMD1_CMD_Command/Compare To Constant
      mask TypeOptions relop: == | ~= | < | <= | >= | >
      mask TypeOptions OutDataTypeStr: Simulink:masks:uint8 | Simulink:masks:boolean
      mask Callback ZeroCross: sl('zeroCrossEnable', gcbh);
      mask Display: disp(str)
  Compare To Constant1 : Subsystem  mask(Compare To Constant){relop===, const=1, OutDataTypeStr=boolean, ZeroCross=on}
      mask prompts: relop "Simulink:masks:Operator_MP"; const "Simulink:masks:ConstantValue_MP"; OutDataTypeStr "Simulink:masks:OutputDataType_MP"; ZeroCross "Simulink:masks:EnableZerocrossingDetection_MP"
      mask help: Simulink:masks:CompareToConstant_MD
      mask init: same as Enrg_conv_El_to_Mec_Bosch/PTI_DriveEmot_Bosch/EMD1_CMD_Command/Compare To Constant
      mask TypeOptions relop: == | ~= | < | <= | >= | >
      mask TypeOptions OutDataTypeStr: Simulink:masks:uint8 | Simulink:masks:boolean
      mask Callback ZeroCross: sl('zeroCrossEnable', gcbh);
      mask Display: disp(str)
  Constant : Constant  Value=4
  Constant3 : Constant
  Constant4 : Constant  Value=0
  Switch : Switch  Threshold=0.5
  Switch1 : Switch  Threshold=0.5
  Out_EMD1_CMD_Command : Outport
  wires:
  Compare To Constant/1(y) -> Switch1/2
  Switch/1 -> Out_EMD1_CMD_Command/1
  Constant4/1 -> Switch1/3
  Constant3/1 -> Switch1/1
  Constant/1 -> Switch/1
  Switch1/1 -> Switch/3
  Compare To Constant1/1(y) -> Switch/2
  EMD1_CMD_ClearErrors/1 -> Compare To Constant1/1(u)
  EMD1_CMD_MotorControlMode/1 -> Compare To Constant/1(u)

== system Enrg_conv_El_to_Mec_Bosch/PTI_DriveEmot_Bosch/EMD1_CMD_Command3 ==
  EMD1_CMD_ClearErrors : Inport
  EMD1_CMD_MotorControlMode : Inport  Port=2
  Compare To Constant : Subsystem  mask(Compare To Constant){relop===, const=1, OutDataTypeStr=boolean, ZeroCross=on}
      mask prompts: relop "Simulink:masks:Operator_MP"; const "Simulink:masks:ConstantValue_MP"; OutDataTypeStr "Simulink:masks:OutputDataType_MP"; ZeroCross "Simulink:masks:EnableZerocrossingDetection_MP"
      mask help: Simulink:masks:CompareToConstant_MD
      mask init: same as Enrg_conv_El_to_Mec_Bosch/PTI_DriveEmot_Bosch/EMD1_CMD_Command/Compare To Constant
      mask TypeOptions relop: == | ~= | < | <= | >= | >
      mask TypeOptions OutDataTypeStr: Simulink:masks:uint8 | Simulink:masks:boolean
      mask Callback ZeroCross: sl('zeroCrossEnable', gcbh);
      mask Display: disp(str)
  Compare To Constant1 : Subsystem  mask(Compare To Constant){relop===, const=1, OutDataTypeStr=boolean, ZeroCross=on}
      mask prompts: relop "Simulink:masks:Operator_MP"; const "Simulink:masks:ConstantValue_MP"; OutDataTypeStr "Simulink:masks:OutputDataType_MP"; ZeroCross "Simulink:masks:EnableZerocrossingDetection_MP"
      mask help: Simulink:masks:CompareToConstant_MD
      mask init: same as Enrg_conv_El_to_Mec_Bosch/PTI_DriveEmot_Bosch/EMD1_CMD_Command/Compare To Constant
      mask TypeOptions relop: == | ~= | < | <= | >= | >
      mask TypeOptions OutDataTypeStr: Simulink:masks:uint8 | Simulink:masks:boolean
      mask Callback ZeroCross: sl('zeroCrossEnable', gcbh);
      mask Display: disp(str)
  Constant : Constant  Value=4
  Constant3 : Constant
  Constant4 : Constant  Value=0
  Switch : Switch  Threshold=0.5
  Switch1 : Switch  Threshold=0.5
  Out_EMD1_CMD_Command : Outport
  wires:
  Compare To Constant/1(y) -> Switch1/2
  Switch/1 -> Out_EMD1_CMD_Command/1
  Constant4/1 -> Switch1/3
  Constant3/1 -> Switch1/1
  Constant/1 -> Switch/1
  Switch1/1 -> Switch/3
  Compare To Constant1/1(y) -> Switch/2
  EMD1_CMD_ClearErrors/1 -> Compare To Constant1/1(u)
  EMD1_CMD_MotorControlMode/1 -> Compare To Constant/1(u)

== system Enrg_conv_El_to_Mec_Bosch/PTI_DriveEmot_Bosch/Emot1_4 ==
  emot_Emot1_angVel : Inport
  voltBatHV1 : Inport  Port=2
  trqEmotDesPhy1 : Inport  Port=3
  voltBatHV4 : Inport  Port=4
  trqEmotDesPhy4 : Inport  Port=5
  drvEmot1_Oil_Temperature : Inport  Port=6
  drvEmot1_Coolant_Temperature : Inport  Port=7
  drvEmot_Ambient_Temperature : Inport  Port=8
  inv_coolant_temperature : Inport  Port=9
  inv1_switching_freq : Inport  Port=10
  inv4_switching_freq : Inport  Port=11
  emot_Emot4_angVel : Inport  Port=12
  drvEmot4_Oil_Temperature : Inport  Port=13
  drvEmot4_Coolant_Temperature : Inport  Port=14
  Emot1_Selection : Inport  Port=15
  Emot4_Selection : Inport  Port=16
  drvEmot1CoolantFlow_vdot : Inport  Port=17
  drvEmot1OilFlow_vdot : Inport  Port=18
  driveInverterCoolantFlow_vdot : Inport  Port=19
  drvEmot4CoolantFlow_vdot : Inport  Port=20
  drvEmot4OilFlow_vdot : Inport  Port=21
  Bus Creator1 : BusCreator  Inputs=17
  Bus Creator2 : BusCreator  Inputs=17
  Bus Creator3 : BusCreator  Inputs=2
  e-Motor1 Bosch : Enrg_conv_El_to_Mec_Bosch/e-Motor Bosch  SystemSampleTime=-1
  e-Motor4 Bosch : Enrg_conv_El_to_Mec_Bosch/e-Motor Bosch  SystemSampleTime=-1
  emot1_4B : Outport
  wires:
  drvEmot1_Oil_Temperature/1 -> e-Motor1 Bosch/4
  inv_coolant_temperature/1 -> e-Motor4 Bosch/7, e-Motor1 Bosch/7
  e-Motor1 Bosch/1 -> Bus Creator1/1  "pwrEmotPhy"
  emot_Emot1_angVel/1 -> e-Motor1 Bosch/1
  trqEmotDesPhy1/1 -> e-Motor1 Bosch/3
  voltBatHV1/1 -> e-Motor1 Bosch/2
  emot_Emot4_angVel/1 -> e-Motor4 Bosch/1
  voltBatHV4/1 -> e-Motor4 Bosch/2
  Bus Creator1/1 -> Bus Creator3/1  "emot1B"
  Bus Creator2/1 -> Bus Creator3/2  "emot4B"
  trqEmotDesPhy4/1 -> e-Motor4 Bosch/3
  Bus Creator3/1 -> emot1_4B/1  "emot1_4B"
  Emot4_Selection/1 -> e-Motor4 Bosch/Enable
  Emot1_Selection/1 -> e-Motor1 Bosch/Enable
  drvEmot4_Oil_Temperature/1 -> e-Motor4 Bosch/4
  drvEmot1_Coolant_Temperature/1 -> e-Motor1 Bosch/5
  drvEmot_Ambient_Temperature/1 -> e-Motor4 Bosch/6, e-Motor1 Bosch/6
  inv1_switching_freq/1 -> e-Motor1 Bosch/8
  drvEmot4_Coolant_Temperature/1 -> e-Motor4 Bosch/5
  e-Motor1 Bosch/13 -> Bus Creator1/13  "iStator"
  e-Motor1 Bosch/9 -> Bus Creator1/9  "driveInverter_wasteHeat_power"
  e-Motor1 Bosch/10 -> Bus Creator1/10  "driveInverter_Temperatures"
  e-Motor1 Bosch/8 -> Bus Creator1/8  "drvEmot_T_Stator"
  e-Motor1 Bosch/7 -> Bus Creator1/7  "drvEmot_wasteHeat_power"
  e-Motor1 Bosch/6 -> Bus Creator1/6  "trqEmotMax"
  e-Motor1 Bosch/3 -> Bus Creator1/3  "Inv_Ploss"
  e-Motor1 Bosch/5 -> Bus Creator1/5  "trqEmotPhy"
  e-Motor1 Bosch/4 -> Bus Creator1/4  "mot_Ploss"
  e-Motor1 Bosch/11 -> Bus Creator1/11  "drvEmot_T_Rotor"
  e-Motor1 Bosch/12 -> Bus Creator1/12  "uStator"
  e-Motor1 Bosch/2 -> Bus Creator1/2  "iDcInverter"
  e-Motor4 Bosch/1 -> Bus Creator2/1  "pwrEmotPhy"
  e-Motor4 Bosch/13 -> Bus Creator2/13  "iStator"
  e-Motor4 Bosch/9 -> Bus Creator2/9  "driveInverter_wasteHeat_power"
  e-Motor4 Bosch/10 -> Bus Creator2/10  "driveInverter_Temperatures"
  e-Motor4 Bosch/8 -> Bus Creator2/8  "drvEmot_T_Stator"
  e-Motor4 Bosch/7 -> Bus Creator2/7  "drvEmot_wasteHeat_power"
  e-Motor4 Bosch/6 -> Bus Creator2/6  "trqEmotMax"
  e-Motor4 Bosch/3 -> Bus Creator2/3  "Inv_Ploss"
  e-Motor4 Bosch/5 -> Bus Creator2/5  "trqEmotPhy"
  e-Motor4 Bosch/4 -> Bus Creator2/4  "mot_Ploss"
  e-Motor4 Bosch/11 -> Bus Creator2/11  "drvEmot_T_Rotor"
  e-Motor4 Bosch/12 -> Bus Creator2/12  "uStator"
  e-Motor4 Bosch/2 -> Bus Creator2/2  "iDcInverter"
  e-Motor1 Bosch/14 -> Bus Creator1/14  "modIdx"
  e-Motor1 Bosch/15 -> Bus Creator1/15  "cosPhi"
  e-Motor4 Bosch/14 -> Bus Creator2/14  "modIdx"
  e-Motor4 Bosch/15 -> Bus Creator2/15  "cosPhi"
  inv4_switching_freq/1 -> e-Motor4 Bosch/8
  drvEmot1CoolantFlow_vdot/1 -> e-Motor1 Bosch/9
  drvEmot1OilFlow_vdot/1 -> e-Motor1 Bosch/10
  driveInverterCoolantFlow_vdot/1 -> e-Motor4 Bosch/11, e-Motor1 Bosch/11
  drvEmot4OilFlow_vdot/1 -> e-Motor4 Bosch/10
  drvEmot4CoolantFlow_vdot/1 -> e-Motor4 Bosch/9
  e-Motor1 Bosch/16 -> Bus Creator1/16  "wasteHeat_coolant"
  e-Motor1 Bosch/17 -> Bus Creator1/17  "wasteHeat_oil"
  e-Motor4 Bosch/16 -> Bus Creator2/16  "wasteHeat_coolant"
  e-Motor4 Bosch/17 -> Bus Creator2/17  "wasteHeat_oil"

== system Enrg_conv_El_to_Mec_Bosch/PTI_DriveEmot_Bosch/Emot2_3 ==
  emot_Emot2_angVel : Inport
  voltBatHV2 : Inport  Port=2
  trqEmotDesPhy2 : Inport  Port=3
  voltBatHV3 : Inport  Port=4
  trqEmotDesPhy3 : Inport  Port=5
  drvEmot2_Oil_Temperature : Inport  Port=6
  drvEmot2_Coolant_Temperature : Inport  Port=7
  drvEmot_Ambient_Temperature : Inport  Port=8
  inv_coolant_temperature : Inport  Port=9
  inv2_switching_freq : Inport  Port=10
  inv3_switching_freq : Inport  Port=11
  emot_Emot3_angVel : Inport  Port=12
  drvEmot3_Oil_Temperature : Inport  Port=13
  drvEmot3_Coolant_Temperature : Inport  Port=14
  Emot2_Selection : Inport  Port=15
  Emot3_Selection : Inport  Port=16
  drvEmot2CoolantFlow_vdot : Inport  Port=17
  drvEmot2OilFlow_vdot : Inport  Port=18
  driveInverterCoolantFlow_vdot : Inport  Port=19
  drvEmot3CoolantFlow_vdot : Inport  Port=20
  drvEmot3OilFlow_vdot : Inport  Port=21
  Bus Creator1 : BusCreator  Inputs=17
  Bus Creator2 : BusCreator  Inputs=17
  Bus Creator3 : BusCreator  Inputs=2
  e-Motor2 Bosch : Enrg_conv_El_to_Mec_Bosch/e-Motor Bosch  SystemSampleTime=-1
  e-Motor3 Bosch : Enrg_conv_El_to_Mec_Bosch/e-Motor Bosch  SystemSampleTime=-1
  emot2_3B : Outport
  wires:
  Bus Creator3/1 -> emot2_3B/1  "emot2_3B"
  Bus Creator1/1 -> Bus Creator3/1  "emot2B"
  drvEmot2_Oil_Temperature/1 -> e-Motor2 Bosch/4
  inv_coolant_temperature/1 -> e-Motor3 Bosch/7, e-Motor2 Bosch/7
  emot_Emot2_angVel/1 -> e-Motor2 Bosch/1
  trqEmotDesPhy2/1 -> e-Motor2 Bosch/3
  voltBatHV2/1 -> e-Motor2 Bosch/2
  Emot2_Selection/1 -> e-Motor2 Bosch/Enable
  drvEmot2_Coolant_Temperature/1 -> e-Motor2 Bosch/5
  drvEmot_Ambient_Temperature/1 -> e-Motor3 Bosch/6, e-Motor2 Bosch/6
  inv2_switching_freq/1 -> e-Motor2 Bosch/8
  emot_Emot3_angVel/1 -> e-Motor3 Bosch/1
  voltBatHV3/1 -> e-Motor3 Bosch/2
  trqEmotDesPhy3/1 -> e-Motor3 Bosch/3
  drvEmot3_Oil_Temperature/1 -> e-Motor3 Bosch/4
  drvEmot3_Coolant_Temperature/1 -> e-Motor3 Bosch/5
  Bus Creator2/1 -> Bus Creator3/2  "emot3B"
  Emot3_Selection/1 -> e-Motor3 Bosch/Enable
  e-Motor2 Bosch/1 -> Bus Creator1/1  "pwrEmotPhy"
  e-Motor2 Bosch/13 -> Bus Creator1/13  "iStator"
  e-Motor2 Bosch/9 -> Bus Creator1/9  "driveInverter_wasteHeat_power"
  e-Motor2 Bosch/10 -> Bus Creator1/10  "driveInverter_Temperatures"
  e-Motor2 Bosch/8 -> Bus Creator1/8  "drvEmot_T_Stator"
  e-Motor2 Bosch/7 -> Bus Creator1/7  "drvEmot_wasteHeat_power"
  e-Motor2 Bosch/6 -> Bus Creator1/6  "trqEmotMax"
  e-Motor2 Bosch/3 -> Bus Creator1/3  "Inv_Ploss"
  e-Motor2 Bosch/5 -> Bus Creator1/5  "trqEmotPhy"
  e-Motor2 Bosch/4 -> Bus Creator1/4  "mot_Ploss"
  e-Motor2 Bosch/11 -> Bus Creator1/11  "drvEmot_T_Rotor"
  e-Motor2 Bosch/12 -> Bus Creator1/12  "uStator"
  e-Motor2 Bosch/2 -> Bus Creator1/2  "iDcInverter"
  e-Motor2 Bosch/14 -> Bus Creator1/14  "modIdx"
  e-Motor2 Bosch/15 -> Bus Creator1/15  "cosPhi"
  e-Motor3 Bosch/1 -> Bus Creator2/1  "pwrEmotPhy"
  e-Motor3 Bosch/13 -> Bus Creator2/13  "iStator"
  e-Motor3 Bosch/9 -> Bus Creator2/9  "driveInverter_wasteHeat_power"
  e-Motor3 Bosch/10 -> Bus Creator2/10  "driveInverter_Temperatures"
  e-Motor3 Bosch/8 -> Bus Creator2/8  "drvEmot_T_Stator"
  e-Motor3 Bosch/7 -> Bus Creator2/7  "drvEmot_wasteHeat_power"
  e-Motor3 Bosch/6 -> Bus Creator2/6  "trqEmotMax"
  e-Motor3 Bosch/3 -> Bus Creator2/3  "Inv_Ploss"
  e-Motor3 Bosch/5 -> Bus Creator2/5  "trqEmotPhy"
  e-Motor3 Bosch/4 -> Bus Creator2/4  "mot_Ploss"
  e-Motor3 Bosch/11 -> Bus Creator2/11  "drvEmot_T_Rotor"
  e-Motor3 Bosch/12 -> Bus Creator2/12  "uStator"
  e-Motor3 Bosch/2 -> Bus Creator2/2  "iDcInverter"
  e-Motor3 Bosch/14 -> Bus Creator2/14  "modIdx"
  e-Motor3 Bosch/15 -> Bus Creator2/15  "cosPhi"
  inv3_switching_freq/1 -> e-Motor3 Bosch/8
  drvEmot2CoolantFlow_vdot/1 -> e-Motor2 Bosch/9
  drvEmot2OilFlow_vdot/1 -> e-Motor2 Bosch/10
  driveInverterCoolantFlow_vdot/1 -> e-Motor3 Bosch/11, e-Motor2 Bosch/11
  drvEmot3CoolantFlow_vdot/1 -> e-Motor3 Bosch/9
  drvEmot3OilFlow_vdot/1 -> e-Motor3 Bosch/10
  e-Motor2 Bosch/16 -> Bus Creator1/16  "wasteHeat_coolant"
  e-Motor2 Bosch/17 -> Bus Creator1/17  "wasteHeat_oil"
  e-Motor3 Bosch/16 -> Bus Creator2/16  "wasteHeat_coolant"
  e-Motor3 Bosch/17 -> Bus Creator2/17  "wasteHeat_oil"

== system Enrg_conv_El_to_Mec_Bosch/PTI_DriveEmot_Bosch/MotorSelection ==
  MidAxle : Constant  Value=FirstDrivenAxle_FirstDrivenAxleNoOfEmot
  RearAxle : Constant  Value=SecondDrivenAxle_SecondDrivenAxleNoOfEmot
  Truth Table : Truth Table  TreatAsAtomicUnit=on
  Emot1_Selection : Outport
  Emot2_Selection : Outport  Port=2
  Emot3_Selection : Outport  Port=3
  Emot4_Selection : Outport  Port=4
  wires:
  MidAxle/1 -> Truth Table/1(u1)
  RearAxle/1 -> Truth Table/2(u2)
  Truth Table/1(y1) -> Emot1_Selection/1
  Truth Table/2(y2) -> Emot2_Selection/1
  Truth Table/3(y3) -> Emot3_Selection/1
  Truth Table/4(y4) -> Emot4_Selection/1
